simulink model "Single_shunt_sampling"  (R2025a)
settings: Solver=FixedStepAuto  StartTime=0.0  StopTime=2  FixedStep=0.00001  RelTol=1e-3
InitFcn:
  | We_Speed = 900;
  | Unobservable = 0.7; % (0-0.866)
  | zeta = 0.05;
settings Model: Creator=星必尘Sguan  LastModifiedBy=星必尘Sguan

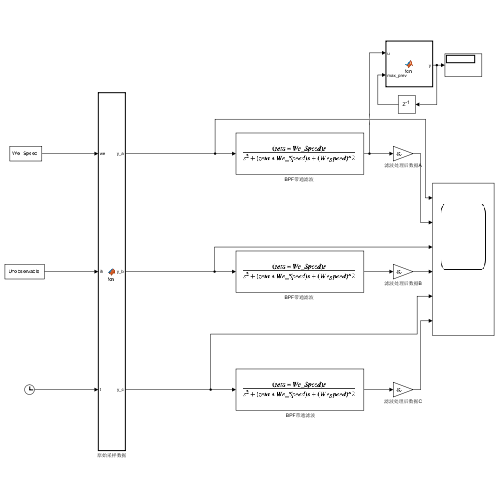
[thumbnail: Simulink's stored preview of the top-level diagram]
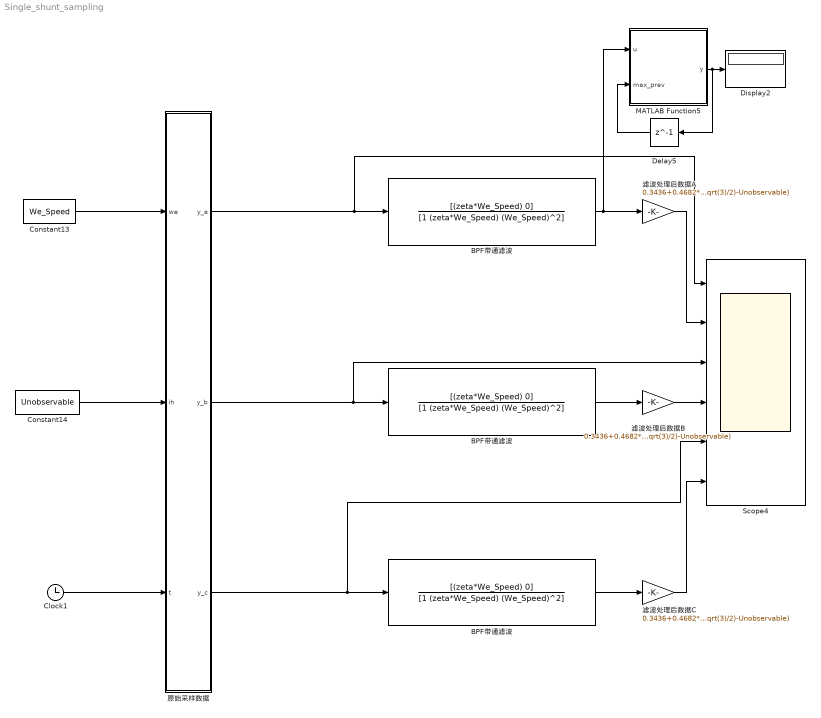
== system Single_shunt_sampling ==
  "     BPF带通滤波    " : TransferFcn  Numerator=[(zeta*We_Speed) 0]  Denominator=[1 (zeta*We_Speed) (We_Speed)^2]
  "  BPF带通滤波   " : TransferFcn  Numerator=[(zeta*We_Speed) 0]  Denominator=[1 (zeta*We_Speed) (We_Speed)^2]
  "BPF带通滤波 " : TransferFcn  Numerator=[(zeta*We_Speed) 0]  Denominator=[1 (zeta*We_Speed) (We_Speed)^2]
  Clock1 : Clock
  Constant13 : Constant  Value=We_Speed
  Constant14 : Constant  Value=Unobservable
  Delay5 : Delay  DelayLength=1  InputProcessing=Columns as channels (frame based)
  Display2 : Display
  MATLAB Function5 : MATLAB Function  TreatAsAtomicUnit=on
  Scope4 : Scope  NumInputPorts=6
      settings: ActiveDisplayYMinimum=-1.2499999999775429  ActiveDisplayYMaximum=1.2499999999852798  DataLoggingVariableName=ScopeData22
  原始采样数据 : MATLAB Function  TreatAsAtomicUnit=on
  滤波处理后数据A : Gain  Gain=0.3436+0.4682*Unobservable+0.5278/((sqrt(3)/2)-Unobservable)
  滤波处理后数据B : Gain  Gain=0.3436+0.4682*Unobservable+0.5278/((sqrt(3)/2)-Unobservable)
  滤波处理后数据C : Gain  Gain=0.3436+0.4682*Unobservable+0.5278/((sqrt(3)/2)-Unobservable)
  wires:
  滤波处理后数据C/1 -> Scope4/6
  原始采样数据/2(y_b) -> Scope4/3, "  BPF带通滤波   "/1
  原始采样数据/3(y_c) -> Scope4/5, "     BPF带通滤波    "/1
  "  BPF带通滤波   "/1 -> 滤波处理后数据B/1
  滤波处理后数据B/1 -> Scope4/4
  "     BPF带通滤波    "/1 -> 滤波处理后数据C/1
  原始采样数据/1(y_a) -> Scope4/1, "BPF带通滤波 "/1
  Delay5/1 -> MATLAB Function5/2(max_prev)
  MATLAB Function5/1(y) -> Delay5/1, Display2/1
  Clock1/1 -> 原始采样数据/3(t)
  "BPF带通滤波 "/1 -> 滤波处理后数据A/1, MATLAB Function5/1(u)
  Constant14/1 -> 原始采样数据/2(ih)
  Constant13/1 -> 原始采样数据/1(we)
  滤波处理后数据A/1 -> Scope4/2

== matlab function Single_shunt_sampling/原始采样数据 ==
  data: we input; y_a output; ih input; t input; y_b output; y_c output
function [y_a, y_b, y_c] = fcn(we, ih, t)
%#codegen
% 输入：
%   we - 角频率 (rad/s)
%   ih - 不可观测区参数 (0 ~ sqrt(3)/2)，决定归零区间宽度
%   t  - 仿真时间 (s)，从 Clock 模块输入
% 输出：
%   y_a, y_b, y_c - 修正后的三相正弦波（各相隔120°，每个波形在60°整数倍点左侧归零）

% -------- 参数限幅 --------
ih_max = sqrt(3)/2;
ih_limited = min(abs(ih), ih_max);

% -------- 归零宽度：asin(ih) 弧度，转为角度 --------
zero_width_deg = asin(ih_limited) * 180 / pi;  % 0° ~ 60°

% -------- 计算三个相位的角度（弧度） --------
theta_a = mod(we * t, 2*pi);
theta_b = mod(theta_a - 2*pi/3, 2*pi);  % A相滞后120°
theta_c = mod(theta_a + 2*pi/3, 2*pi);  % A相超前120°

% -------- 分别计算三个相位的修正波形 --------
y_a = apply_zero_zone(theta_a, zero_width_deg);
y_b = apply_zero_zone(theta_b, zero_width_deg);
y_c = apply_zero_zone(theta_c, zero_width_deg);

end

% -------- 子函数：对单个角度应用归零处理 --------
function y = apply_zero_zone(theta, zero_width_deg)
    % 将弧度转为角度
    theta_deg = theta * 180 / pi;
    
    % 在60°周期内的位置 (0~60°)
    pos_in_60deg = mod(theta_deg, 60);
    
    % 判断：在60°整数倍点的左侧 [60-width, 60) 区间归零
    if pos_in_60deg >= (60 - zero_width_deg) && pos_in_60deg < 60
        y = 0;
    else
        y = sin(theta);
    end
end

== matlab function Single_shunt_sampling/MATLAB Function5 ==
  data: u input; y output; max_prev input
function y = fcn(u, max_prev)
%#codegen
% 输入：
%   u        - 当前输入数值
%   max_prev - 上一拍的历史最大值（来自 Unit Delay）
% 输出：
%   y        - 新的历史最大值

% 比较当前值和上一拍最大值
if u > max_prev
    y = u;
else
    y = max_prev;
end

end
